simulink model "Implementcion_Adruino"  (R2023b)
settings: Solver=FixedStepAuto  StartTime=0.0  StopTime=inf  RelTol=1e-3  EnableMultiTasking=on
undefined symbols (not defined in the file): betaF, g, J, Kf, Lb, Lm, m_b, m_m
libraries: arduinolib x2, SignalEditorBlockLib x1, simulink_extras x1
settings Model: ExtModeTrigDuration=2  Creator=alfar  LastModifiedBy=chris
settings OptimizationCC: EnhancedBackFolding=on  PassReuseOutputArgsAs=Individual arguments  ZeroExternalMemoryAtStartup=off  ZeroInternalMemoryAtStartup=off  MaxStackSize=64  OptimizeBlockOrder=speed  DifferentSizesBufferReuse=on  OptimizationCustomize=off  EfficientTunableParamExpr=on
settings DebuggingCC: ParameterTunabilityLossMsg=error
settings HardwareCC: ProdBitPerInt=16  ProdBitPerPointer=16  ProdBitPerSizeT=16  ProdBitPerPtrDiffT=16  ProdLargestAtomicFloat=None  ProdWordSize=8  ProdHWDeviceType=Atmel->AVR  UseEmbeddedCoderFeatures=off  UseSimulinkCoderFeatures=off
settings SFSimCC: MATLABDynamicMemAlloc=off
settings RTWCC: Description=Embedded Coder  SystemTargetFile=ert.tlc  HardwareBoard=Arduino Mega 2560  TemplateMakefile=ert_default_tmf  Toolchain=Arduino AVR  BuildConfiguration=Faster Runs  GPUComputeCapability=5.0
settings CodeAppCC: ForceParamTrailComments=on  IgnoreCustomStorageClasses=off  OperatorAnnotations=on  SimulinkDataObjDesc=on  SFDataObjDesc=on  InsertBlockDesc=on
settings ERTTargetCC: SupportContinuousTime=on  SupportNonInlinedSFcns=on  SupportVariableSizeSignals=on  ExtModeTransport=3  ExtModeStaticAlloc=on  ExtModeAutomaticAllocSize=off  ExtModeStaticAllocSize=2048  ExtModeMexFile=ext_xcp  ExtModeIntrfLevel=Level2 - Open

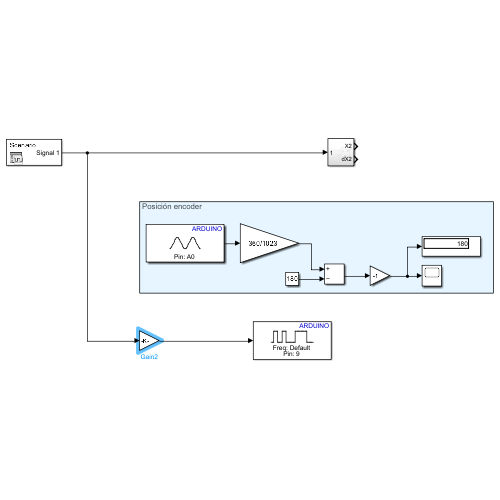
[thumbnail: Simulink's stored preview of the top-level diagram]
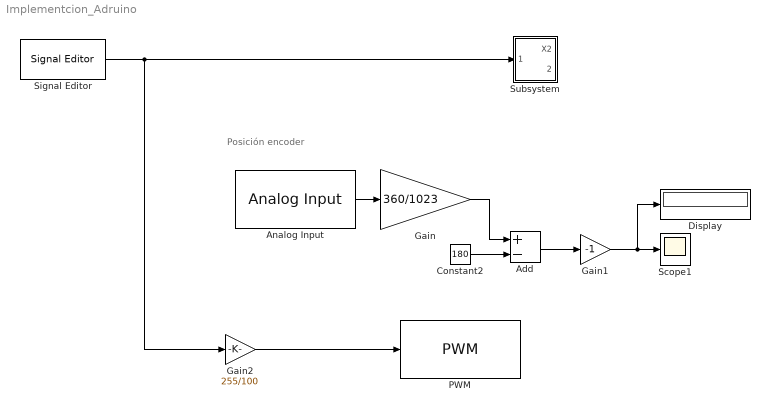
== system Implementcion_Adruino ==
  note: Posición encoder
  Add : Sum  Inputs=+-
  Analog Input : arduinolib/Analog Input  pinNumber=0  ReadResultsOnly=off  ConversionTriggerSource=Software  ExternalTriggerType=uint32( 0 )  OutputDataType=uint16  EnableConversionCompleteNotify=off  EnableOuputStatus=off  SampleTime=-1  blockPlatform=arduino
  Constant2 : Constant  Value=180
  Display : Display
  Gain : Gain  Gain=360/1023
  Gain1 : Gain  Gain=-1
  Gain2 : Gain  Gain=255/100
  PWM : arduinolib/PWM  pinNumber=9  frequencyType=Default  desiredFrequency=490.2  achievableFrequency=490.2
  Scope1 : Scope
  Signal Editor : SignalEditorBlockLib/Signal Editor  FileName=TrenPulsos.mat  ActiveScenario=Scenario  ActiveSignal=Signal 1  IsBus=off  OutputBusObjectStr=Bus: BusObject  SampleTime=0  Interpolate=off  ZeroCross=off  OutputAfterFinalValue=Setting to zero  Unit=inherit  PreserveSignalName=on  ApplySigPropsToAllScenarios=on  ApplySigPropsToAllSignals=off
  Subsystem : Subsystem
  wires:
  Signal Editor/1 -> Gain2/1, Subsystem/1(In1)
  Add/1 -> Gain1/1
  Constant2/1 -> Add/2
  Gain/1 -> Add/1
  Gain1/1 -> Display/1, Scope1/1
  Analog Input/1 -> Gain/1
  Gain2/1 -> PWM/1

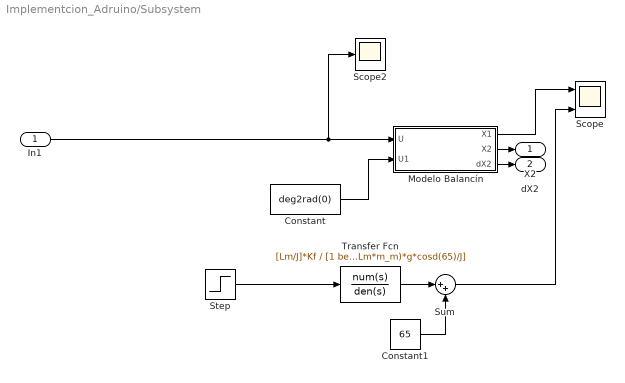
== system Implementcion_Adruino/Subsystem ==
  In1 : Inport
  Constant : Constant  Value=deg2rad(0)
  Constant1 : Constant  Value=65
  Modelo Balancín : Subsystem
  Scope : Scope  NumInputPorts=2
  Scope2 : Scope
  Step : Step  Time=50  After=-15  SampleTime=0
  Sum : Sum  Inputs=|++
  Transfer Fcn : TransferFcn  Numerator=[Lm/J]*Kf  Denominator="[1 betaF/J  (Lb*m_b+Lm*m_m)*g*cosd(65)/J]"
  X2 : Outport
  dX2 : Outport  Port=2
  wires:
  Sum/1 -> Scope/2
  Modelo Balancín/1(X1) -> Scope/1
  Constant1/1 -> Sum/2
  Transfer Fcn/1 -> Sum/1
  Constant/1 -> Modelo Balancín/2(U1)
  In1/1 -> Scope2/1, Modelo Balancín/1(U)
  Step/1 -> Transfer Fcn/1
  Modelo Balancín/2(X2) -> X2/1
  Modelo Balancín/3(dX2) -> dX2/1

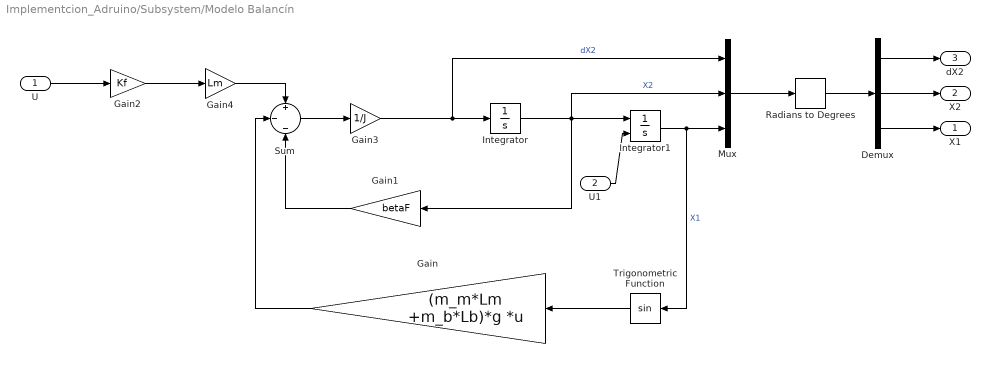
== system Implementcion_Adruino/Subsystem/Modelo Balancín ==
  U : Inport
  U1 : Inport  Port=2
  Demux : Demux  Outputs=3
  Gain : Gain  Gain=(m_m*Lm +m_b*Lb)*g  Multiplication=Matrix(K*u)
  Gain1 : Gain  Gain=betaF
  Gain2 : Gain  Gain=Kf
  Gain3 : Gain  Gain=1/J
  Gain4 : Gain  Gain=Lm
  Integrator : Integrator
  Integrator1 : Integrator  InitialConditionSource=external  InitialCondition=80*pi/180
  Mux : Mux  Inputs=3
  Radians to Degrees : simulink_extras/Transformations/Radians to Degrees
  Sum : Sum  Inputs=+|-|-
  Trigonometric Function : Trigonometry
  X1 : Outport
  X2 : Outport  Port=2
  dX2 : Outport  Port=3
  wires:
  Integrator/1 -> Mux/2, Integrator1/1, Gain1/1  "X2"
  Gain3/1 -> Mux/1, Integrator/1  "dX2"
  Trigonometric Function/1 -> Gain/1
  Mux/1 -> Radians to Degrees/1
  Gain/1 -> Sum/2
  Radians to Degrees/1 -> Demux/1
  Sum/1 -> Gain3/1
  Gain1/1 -> Sum/3
  Gain2/1 -> Gain4/1
  Integrator1/1 -> Mux/3, Trigonometric Function/1  "X1"
  U/1 -> Gain2/1
  U1/1 -> Integrator1/2
  Demux/1 -> dX2/1
  Demux/2 -> X2/1
  Demux/3 -> X1/1
  Gain4/1 -> Sum/1
